simulink model "Amplitude_Shift_Keying"  (R2015a)
settings: Solver=ode45  StartTime=0.0  StopTime=10.0  RelTol=1e-3
settings Model: Creator=Chayti  LastModifiedBy=hp

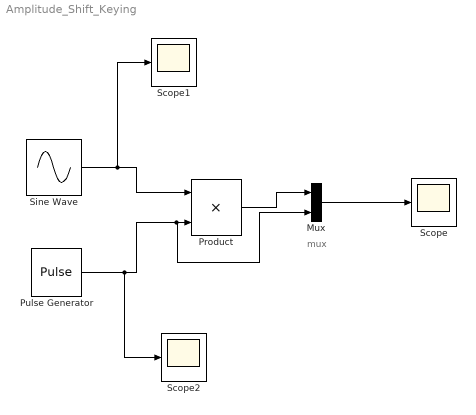
== system Amplitude_Shift_Keying ==
  note: mux
  Mux : Mux  Inputs=2
  Product : Product
  Pulse Generator : DiscretePulseGenerator  PulseType=Time based  PulseWidth=50
  Scope : Scope
  Scope1 : Scope
  Scope2 : Scope
      settings: SaveName=ScopeData2
  Sine Wave : Sin  Amplitude=-2  Frequency=100  SampleTime=0.001
  wires:
  Sine Wave/1 -> Scope1/1, Product/1
  Mux/1 -> Scope/1
  Product/1 -> Mux/1
  Pulse Generator/1 -> Scope2/1, Mux/2, Product/2
